simulink model "ROSCO"  (R2023a)
settings: Solver=ode4  StartTime=0.0  StopTime=TMax  FixedStep=simu.dt  RelTol=1e-3  EnableMultiTasking=on
undefined symbols (not defined in the file): A_total, Azimuth_list, B_total, Bd_total, C_total, D_total, Dd_total, DiscIntNeverNeededParam, F, n_FixFrameInputs, n_FixFrameOutputs, n_FixFrameStates2, n_RotTripletInputs, n_RotTripletOutputs, n_RotTripletStates2, new_seq_inp, new_seq_out, new_seq_states, OutList, Parameter, R, rpm2radps, simu, strmatch, uop_total, windspeed_list, wop_total, xop_total, yop_List_total
libraries: simulink x10
(part 2 of 5)

== system ROSCO/LinearModel_Simulink/Transverseu ==
  Azimuth : Inport
  delta_u : Inport  Port=2
  new_seq_inp : Inport  Port=3
  Constant7 : Constant  Value=n_FixFrameInputs
  Constant8 : Constant  Value=n_RotTripletInputs
  MATLAB Function : MATLAB Function  TreatAsAtomicUnit=on
  delta_u_dq : Outport
  wires:
  Constant8/1 -> MATLAB Function/3(n_RotTripletInputs)
  Azimuth/1 -> MATLAB Function/1(Azimuth)
  Constant7/1 -> MATLAB Function/2(n_FixFrameInputs)
  delta_u/1 -> MATLAB Function/4(delta_u)
  new_seq_inp/1 -> MATLAB Function/5(new_seq_inp)
  MATLAB Function/1(delat_u_dq) -> delta_u_dq/1

== system ROSCO/LinearModel_Simulink/uop2uop_dq ==
  Azimuth : Inport
  uop : Inport  Port=2
  Constant1 : Constant  Value=new_seq_inp
  Constant7 : Constant  Value=n_FixFrameInputs
  Constant8 : Constant  Value=n_RotTripletInputs
  MATLAB Function1 : MATLAB Function  TreatAsAtomicUnit=on
  uop_dq : Outport
  wires:
  Constant7/1 -> MATLAB Function1/2(n_FixFrameInputs)
  uop/1 -> MATLAB Function1/4(u)
  MATLAB Function1/1(u_dq) -> uop_dq/1
  Azimuth/1 -> MATLAB Function1/1(Azimuth)
  Constant1/1 -> MATLAB Function1/5(new_seq_inp)
  Constant8/1 -> MATLAB Function1/3(n_RotTripletInputs)

== system ROSCO/LinearModel_Simulink/y_NonLinear ==
  OutData : Inport
  Extract GenSpeed : Fcn  Expr=u(strmatch('GenSpeed',OutList))
  Extract RootMyc1 : Fcn  Expr=u(strmatch('RootMyc1',OutList))
  Extract RootMyc2 : Fcn  Expr=u(strmatch('RootMyc2',OutList))
  Extract RootMyc3 : Fcn  Expr=u(strmatch('RootMyc3',OutList))
  Extract RotSpeed : Fcn  Expr=u(strmatch('RotSpeed',OutList))
  Mux : Mux  Inputs=5
  y_NR : Outport
  wires:
  OutData/1 -> Extract GenSpeed/1, Extract RotSpeed/1, Extract RootMyc2/1, Extract RootMyc3/1, Extract RootMyc1/1
  Extract RootMyc1/1 -> Mux/3
  Mux/1 -> y_NR/1
  Extract RootMyc2/1 -> Mux/4
  Extract RootMyc3/1 -> Mux/5
  Extract GenSpeed/1 -> Mux/1
  Extract RotSpeed/1 -> Mux/2

== system ROSCO/MPC/Extract Azimuth [deg] ==
  OutData : Inport
  Azimut : Scope  NumInputPorts=2
  Extract Azimuth : Fcn  Expr=u(strmatch('Azimuth',OutList))
  Extract RotSpeed : Fcn  Expr=u(strmatch('RotSpeed',OutList))
  Integrator : Integrator
  mod2pi : Fcn  Expr=rem(u, 2*pi)
  rad2deg : Gain  Gain=1/pi*180
  rpm2rad/s : Gain  Gain=pi/30
  Azimuth : Outport
  wires:
  OutData/1 -> Extract RotSpeed/1, Extract Azimuth/1
  rpm2rad/s/1 -> Integrator/1
  mod2pi/1 -> rad2deg/1
  Integrator/1 -> mod2pi/1
  rad2deg/1 -> Azimut/2, Azimuth/1
  Extract RotSpeed/1 -> rpm2rad/s/1
  Extract Azimuth/1 -> Azimut/1

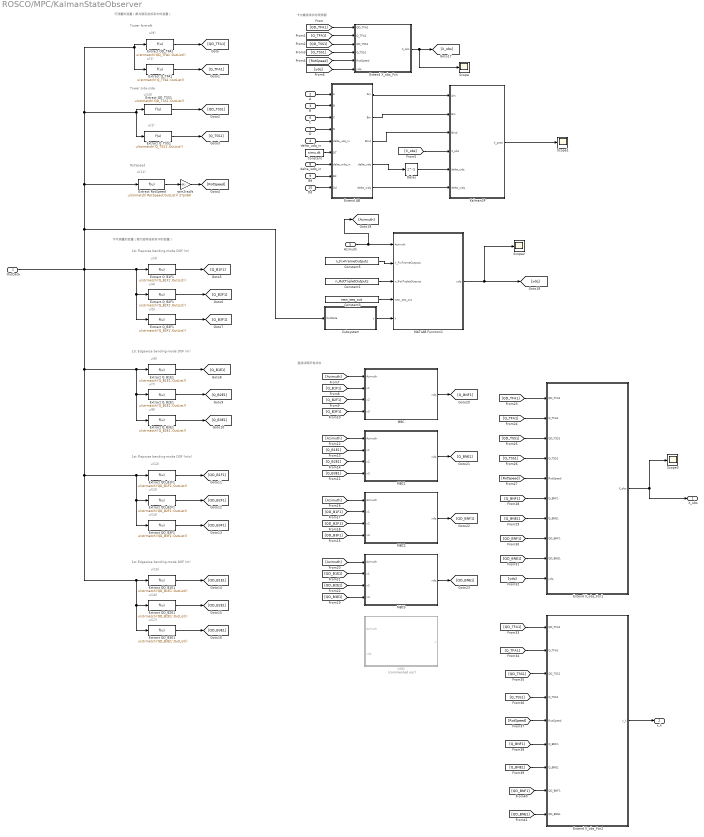
== system ROSCO/MPC/KalmanStateObserver ==
  note: 直接读取所有状态
  note: u(11)
  note: u(2)
  note: u(10)
  note: u(1)
  note: u(9)
  note: 可测量的变量（都为固定坐标系中的变量）
  note: RotSpeed
  note: Tower fore-aft
  note: Tower side-side
  note: 卡尔曼滤波状态观测器
  note: 不可测量的变量（都为旋转坐标系中的变量）
  note: u(3)
  note: u(4)
  note: 1st Flapwise bending-mode DOF (m)
  note: u(5)
  note: u(6)
  note: u(7)
  note: 1st Edgewise bending-mode DOF (m)
  note: u(8)
  note: u(14)
  note: u(12)
  note: u(13)
  note: 1st Flapwise bending-mode DOF (m/s)
  note: 1st Edgewise bending-mode DOF (m)
  note: u(15)
  note: u(17)
  note: u(16)
  OutData : Inport
  A : Inport  Port=2
  B : Inport  Port=3
  delta_udq_in : Inport  Port=4
  Azimuth : Inport  Port=5
  C : Inport  Port=6
  D : Inport  Port=7
  delta_wdq_in : Inport  Port=8
  Bd : Inport  Port=9
  Dd : Inport  Port=10
  Constant : Constant  Value=simu.dt
  Constant1 : Constant  Value=n_RotTripletOutputs
  Constant3 : Constant  Value=new_seq_out
  Constant5 : Constant  Value=n_FixFrameOutputs
  Delay : Delay  DelayLength=1  InitialCondition=0
  Extend AB : MATLAB Function  TreatAsAtomicUnit=on
  Extend X_obs_Fcn : MATLAB Function  TreatAsAtomicUnit=on
  Extend X_obs_Fcn1 : MATLAB Function  TreatAsAtomicUnit=on
  Extend X_obs_Fcn2 : MATLAB Function  TreatAsAtomicUnit=on
  Extract QD_B1E1 : Fcn  Expr=u(strmatch('QD_B1E1',OutList))
  Extract QD_B1F1 : Fcn  Expr=u(strmatch('QD_B1F1',OutList))
  Extract QD_B2E1 : Fcn  Expr=u(strmatch('QD_B2E1',OutList))
  Extract QD_B2F1 : Fcn  Expr=u(strmatch('QD_B2F1',OutList))
  Extract QD_B3E1 : Fcn  Expr=u(strmatch('QD_B3E1',OutList))
  Extract QD_B3F1 : Fcn  Expr=u(strmatch('QD_B3F1',OutList))
  Extract QD_TFA1 : Fcn  Expr=u(strmatch('QD_TFA1',OutList))
  Extract QD_TSS1 : Fcn  Expr=u(strmatch('QD_TSS1',OutList))
  Extract Q_B1E1 : Fcn  Expr=u(strmatch('Q_B1E1',OutList))
  Extract Q_B1F1 : Fcn  Expr=u(strmatch('Q_B1F1',OutList))
  Extract Q_B2E1 : Fcn  Expr=u(strmatch('Q_B2E1',OutList))
  Extract Q_B2F1 : Fcn  Expr=u(strmatch('Q_B2F1',OutList))
  Extract Q_B3E1 : Fcn  Expr=u(strmatch('Q_B3E1',OutList))
  Extract Q_B3F1 : Fcn  Expr=u(strmatch('Q_B3F1',OutList))
  Extract Q_TFA1 : Fcn  Expr=u(strmatch('Q_TFA1',OutList))
  Extract Q_TSS1 : Fcn  Expr=u(strmatch('Q_TSS1',OutList))
  Extract RotSpeed : Fcn  Expr=u(strmatch('RotSpeed',OutList))
  KalmanSP : MATLAB Function  TreatAsAtomicUnit=on
  MATLAB Function1 : MATLAB Function  TreatAsAtomicUnit=on
  MBC : MATLAB Function  TreatAsAtomicUnit=on
  MBC1 : MATLAB Function  TreatAsAtomicUnit=on
  MBC2 : MATLAB Function  TreatAsAtomicUnit=on
  MBC3 : MATLAB Function  TreatAsAtomicUnit=on
  Scope{,1..3} (4 alike) : Scope
  Subsystem : Subsystem
  iMBC : MATLAB Function  Commented=on  TreatAsAtomicUnit=on
  rpm2rad/s : Gain  Gain=2*pi/60
  X_obs : Outport
  x_k : Outport  Port=2
  wires:
  Extract Q_TFA1/1 -> [Q_TFA1]
  Extract QD_TFA1/1 -> [QD_TFA1]
  Extract RotSpeed/1 -> rpm2rad/s/1
  rpm2rad/s/1 -> [RotSpeed]
  Extract QD_TSS1/1 -> [QD_TSS1]
  Extract Q_TSS1/1 -> [Q_TSS1]
  Extract Q_B1F1/1 -> [Q_B1F1]
  Extract Q_B2F1/1 -> [Q_B2F1]
  Extract Q_B3F1/1 -> [Q_B3F1]
  Extract Q_B3E1/1 -> [Q_B3E1]
  Extract Q_B2E1/1 -> [Q_B2E1]
  Extract Q_B1E1/1 -> [Q_B1E1]
  Extract QD_B3F1/1 -> [QD_B3F1]
  Extract QD_B1F1/1 -> [QD_B1F1]
  Extract QD_B2F1/1 -> [QD_B2F1]
  OutData/1 -> Extract QD_TFA1/1, Extract Q_TFA1/1, Extract QD_TSS1/1, Extract Q_TSS1/1, Extract RotSpeed/1, Subsystem/1(OutData), Extract QD_B1E1/1, Extract QD_B2E1/1, Extract QD_B3E1/1, Extract QD_B3F1/1, Extract QD_B2F1/1, Extract QD_B1F1/1, Extract Q_B1E1/1, Extract Q_B2E1/1, Extract Q_B3E1/1, Extract Q_B3F1/1, Extract Q_B2F1/1, Extract Q_B1F1/1
  Extract QD_B3E1/1 -> [QD_B3E1]
  Extract QD_B1E1/1 -> [QD_B1E1]
  Extract QD_B2E1/1 -> [QD_B2E1]
  [QD_TFA1] -> Extend X_obs_Fcn/1(QD_TFA1)
  [Q_TFA1] -> Extend X_obs_Fcn/2(Q_TFA1)
  [QD_TSS1] -> Extend X_obs_Fcn/3(QD_TSS1)
  [Q_TSS1] -> Extend X_obs_Fcn/4(Q_TSS1)
  [RotSpeed] -> Extend X_obs_Fcn/5(RotSpeed)
  Extend X_obs_Fcn/1(X_obs) -> Scope/1, [X_obs]
  [X_obs] -> KalmanSP/4(X_obs)
  Delay/1 -> KalmanSP/5(delta_udq)
  A/1 -> Extend AB/1(A)
  B/1 -> Extend AB/2(B)
  delta_udq_in/1 -> Extend AB/5(delta_udq_in)
  Extend AB/4(delta_udq) -> Delay/1
  Extend AB/2(Bm) -> KalmanSP/2(Bm)
  Extend AB/1(Am) -> KalmanSP/1(Am)
  C/1 -> Extend AB/3(C)
  D/1 -> Extend AB/4(D)
  KalmanSP/1(X_pred) -> Scope1/1
  Subsystem/1(y) -> MATLAB Function1/5(y)
  Constant5/1 -> MATLAB Function1/2(n_FixFrameOutputs)
  Constant1/1 -> MATLAB Function1/3(n_RotTripletOutputs)
  Constant3/1 -> MATLAB Function1/4(new_seq_out)
  Azimuth/1 -> [Azimuth], MATLAB Function1/1(Azimuth)
  MATLAB Function1/1(ydq) -> Scope2/1, [ydq]
  [ydq] -> Extend X_obs_Fcn/6(ydq)
  [Azimuth] -> MBC/1(Azimuth)
  [Q_B1F1] -> MBC/2(x1)
  [Q_B2F1] -> MBC/3(x2)
  [Q_B3F1] -> MBC/4(x3)
  [Q_B3E1] -> MBC1/4(x3)
  [Q_B2E1] -> MBC1/3(x2)
  [Q_B1E1] -> MBC1/2(x1)
  [Azimuth] -> MBC1/1(Azimuth)
  [Azimuth] -> MBC2/1(Azimuth)
  [QD_B1F1] -> MBC2/2(x1)
  [QD_B2F1] -> MBC2/3(x2)
  [QD_B3F1] -> MBC2/4(x3)
  [QD_B3E1] -> MBC3/4(x3)
  [QD_B2E1] -> MBC3/3(x2)
  [QD_B1E1] -> MBC3/2(x1)
  [Azimuth] -> MBC3/1(Azimuth)
  MBC/1(xdq) -> [Q_BNF1]
  MBC1/1(xdq) -> [Q_BNE1]
  MBC2/1(xdq) -> [QD_BNF1]
  MBC3/1(xdq) -> [QD_BNE1]
  [Q_TFA1] -> Extend X_obs_Fcn1/2(Q_TFA1)
  [QD_TSS1] -> Extend X_obs_Fcn1/3(QD_TSS1)
  [RotSpeed] -> Extend X_obs_Fcn1/5(RotSpeed)
  [QD_TFA1] -> Extend X_obs_Fcn1/1(QD_TFA1)
  [Q_TSS1] -> Extend X_obs_Fcn1/4(Q_TSS1)
  [Q_BNF1] -> Extend X_obs_Fcn1/6(Q_BNF1)
  [Q_BNE1] -> Extend X_obs_Fcn1/7(Q_BNE1)
  [QD_BNF1] -> Extend X_obs_Fcn1/8(QD_BNF1)
  [QD_BNE1] -> Extend X_obs_Fcn1/9(QD_BNE1)
  [ydq] -> Extend X_obs_Fcn1/10(ydq)
  Extend X_obs_Fcn1/1(X_obs) -> Scope3/1, X_obs/1
  [QD_TSS1] -> Extend X_obs_Fcn2/3(QD_TSS1)
  [QD_TFA1] -> Extend X_obs_Fcn2/1(QD_TFA1)
  [Q_TSS1] -> Extend X_obs_Fcn2/4(Q_TSS1)
  [QD_BNE1] -> Extend X_obs_Fcn2/9(QD_BNE1)
  [Q_TFA1] -> Extend X_obs_Fcn2/2(Q_TFA1)
  [RotSpeed] -> Extend X_obs_Fcn2/5(RotSpeed)
  [Q_BNF1] -> Extend X_obs_Fcn2/6(Q_BNF1)
  [QD_BNF1] -> Extend X_obs_Fcn2/8(QD_BNF1)
  [Q_BNE1] -> Extend X_obs_Fcn2/7(Q_BNE1)
  Extend X_obs_Fcn2/1(x_k) -> x_k/1
  Constant/1 -> Extend AB/6(DT)
  delta_wdq_in/1 -> Extend AB/7(delta_wdq_in)
  Bd/1 -> Extend AB/8(Bd)
  Dd/1 -> Extend AB/9(Dd)
  Extend AB/3(Bmd) -> KalmanSP/3(Bmd)
  Extend AB/5(delta_wdq) -> KalmanSP/6(delta_wdq)

== system ROSCO/MPC/SwitchOP ==
  WindSpeed : Inport
  MATLAB Function : MATLAB Function  TreatAsAtomicUnit=on
  A : Outport
  B : Outport  Port=2
  C : Outport  Port=3
  D : Outport  Port=4
  yop_list : Outport  Port=5
  xop : Outport  Port=6
  uop : Outport  Port=7
  Bd : Outport  Port=8
  Dd : Outport  Port=9
  wop : Outport  Port=10
  wires:
  WindSpeed/1 -> MATLAB Function/1(windspeed)
  MATLAB Function/1(A) -> A/1
  MATLAB Function/2(B) -> B/1
  MATLAB Function/3(C) -> C/1
  MATLAB Function/4(D) -> D/1
  MATLAB Function/7(yop_list) -> yop_list/1
  MATLAB Function/8(xop) -> xop/1
  MATLAB Function/9(uop) -> uop/1
  MATLAB Function/5(Bd) -> Bd/1
  MATLAB Function/6(Dd) -> Dd/1
  MATLAB Function/10(wop) -> wop/1

== system ROSCO/MPC/Transverseu ==
  Azimuth : Inport
  delta_u : Inport  Port=2
  new_seq_inp : Inport  Port=3
  Constant7 : Constant  Value=n_FixFrameInputs
  Constant8 : Constant  Value=n_RotTripletInputs
  MATLAB Function : MATLAB Function  TreatAsAtomicUnit=on
  delta_u_dq : Outport
  wires:
  Constant8/1 -> MATLAB Function/3(n_RotTripletInputs)
  Azimuth/1 -> MATLAB Function/1(Azimuth)
  Constant7/1 -> MATLAB Function/2(n_FixFrameInputs)
  delta_u/1 -> MATLAB Function/4(delta_u)
  new_seq_inp/1 -> MATLAB Function/5(new_seq_inp)
  MATLAB Function/1(delat_u_dq) -> delta_u_dq/1

== system ROSCO/MPC/y_NonLinear ==
  OutData : Inport
  Extract GenSpeed : Fcn  Expr=u(strmatch('GenSpeed',OutList))
  Extract RootMyc1 : Fcn  Expr=u(strmatch('RootMyc1',OutList))
  Extract RootMyc2 : Fcn  Expr=u(strmatch('RootMyc2',OutList))
  Extract RootMyc3 : Fcn  Expr=u(strmatch('RootMyc3',OutList))
  Extract RotSpeed : Fcn  Expr=u(strmatch('RotSpeed',OutList))
  Mux : Mux  Inputs=5
  y_NR : Outport
  wires:
  OutData/1 -> Extract GenSpeed/1, Extract RotSpeed/1, Extract RootMyc2/1, Extract RootMyc3/1, Extract RootMyc1/1
  Extract RootMyc1/1 -> Mux/3
  Mux/1 -> y_NR/1
  Extract RootMyc2/1 -> Mux/4
  Extract RootMyc3/1 -> Mux/5
  Extract GenSpeed/1 -> Mux/1
  Extract RotSpeed/1 -> Mux/2

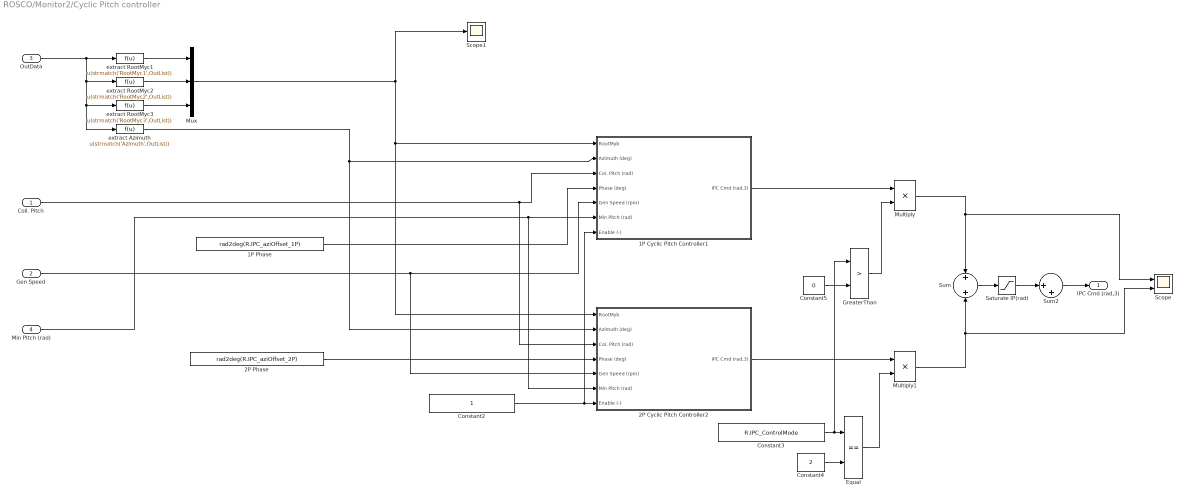
== system ROSCO/Monitor2/Cyclic Pitch controller ==
  Coll. Pitch : Inport
  Gen Speed : Inport  Port=2
  OutData : Inport  Port=3
  Min PItch (rad) : Inport  Port=4
  1P Cyclic Pitch Controller1 : Subsystem
  1P Phase : Constant  Value=rad2deg(R.IPC_aziOffset_1P)
  2P Cyclic Pitch Controller2 : Subsystem
  2P Phase : Constant  Value=rad2deg(R.IPC_aziOffset_2P)
  Constant2 : Constant
  Constant3 : Constant  Value=R.IPC_ControlMode
  Constant4 : Constant  Value=2
  Constant5 : Constant  Value=0
  Equal : RelationalOperator  Operator===  OutDataTypeStr=boolean  RndMeth=Simplest  InputSameDT=off
  GreaterThan : RelationalOperator  Operator=>  OutDataTypeStr=boolean  RndMeth=Simplest  InputSameDT=off
  Multiply : Product
  Multiply1 : Product
  Mux : Mux  Inputs=3
  Saturate IP(rad) : Saturate  UpperLimit=0.052  LowerLimit=-0.052
  Scope : Scope  NumInputPorts=2
  Scope1 : Scope
  Sum : Sum  Inputs=+|+
  Sum2 : Sum  Inputs=|++
  extract Azimuth : Fcn  Expr=u(strmatch('Azimuth',OutList))
  extract RootMyc1 : Fcn  Expr=u(strmatch('RootMyc1',OutList))
  extract RootMyc2 : Fcn  Expr=u(strmatch('RootMyc2',OutList))
  extract RootMyc3 : Fcn  Expr=u(strmatch('RootMyc3',OutList))
  IPC Cmd (rad,3) : Outport  VectorParamsAs1DForOutWhenUnconnected=off
  wires:
  1P Phase/1 -> 1P Cyclic Pitch Controller1/4(Phase (deg))
  Coll. Pitch/1 -> 2P Cyclic Pitch Controller2/3(Col. Pitch (rad)), 1P Cyclic Pitch Controller1/3(Col. Pitch (rad))
  Gen Speed/1 -> 2P Cyclic Pitch Controller2/5(Gen Speed (rpm)), 1P Cyclic Pitch Controller1/5(Gen Speed (rpm))
  1P Cyclic Pitch Controller1/1(IPC Cmd (rad,3)) -> Multiply/1
  Mux/1 -> Scope1/1, 1P Cyclic Pitch Controller1/1(RootMyb), 2P Cyclic Pitch Controller2/1(RootMyb)
  extract Azimuth/1 -> 2P Cyclic Pitch Controller2/2(Azimuth (deg)), 1P Cyclic Pitch Controller1/2(Azimuth (deg))
  Min PItch (rad)/1 -> 2P Cyclic Pitch Controller2/6(Min Pitch (rad)), 1P Cyclic Pitch Controller1/6(Min Pitch (rad))
  2P Phase/1 -> 2P Cyclic Pitch Controller2/4(Phase (deg))
  2P Cyclic Pitch Controller2/1(IPC Cmd (rad,3)) -> Multiply1/1
  Multiply1/1 -> Scope/2, Sum/2
  Multiply/1 -> Sum/1, Scope/1
  Sum/1 -> Saturate IP(rad)/1
  Sum2/1 -> IPC Cmd (rad,3)/1
  Constant2/1 -> 1P Cyclic Pitch Controller1/7(Enable (-)), 2P Cyclic Pitch Controller2/7(Enable (-))
  Constant4/1 -> Equal/2
  Equal/1 -> Multiply1/2
  Constant3/1 -> GreaterThan/1, Equal/1
  Constant5/1 -> GreaterThan/2
  GreaterThan/1 -> Multiply/2
  extract RootMyc2/1 -> Mux/2
  extract RootMyc3/1 -> Mux/3
  OutData/1 -> extract RootMyc1/1, extract RootMyc2/1, extract Azimuth/1, extract RootMyc3/1
  extract RootMyc1/1 -> Mux/1
  Saturate IP(rad)/1 -> Sum2/1

== system ROSCO/PitchSaturation/Integral ==
  x : Inport
  Gain : Inport  Port=2
  Gain1 : Gain  Gain=simu.dt
  Maximum Pitch : Constant  Value=100
  Minimum Pitch : Constant  Value=-100
  Multiply : Product
  Saturate Integral Term : simulink/Discontinuities/Saturation Dynamic  OutMin=[]  OutMax=[]  OutDataTypeStr=Inherit: Same as second input  OutDataType=fixdt(1, 16)  OutScaling=2^-10  RndMeth=Nearest  DoSatur=off
  Scope : Scope  NumInputPorts=2
  Sum : Sum  Inputs=|++
  Unit Delay : UnitDelay  SampleTime=-1  HasFrameUpgradeWarning=on
  Int x : Outport  VectorParamsAs1DForOutWhenUnconnected=off
  wires:
  Maximum Pitch/1 -> Saturate Integral Term/1
  Unit Delay/1 -> Sum/2
  Minimum Pitch/1 -> Saturate Integral Term/3
  Sum/1 -> Saturate Integral Term/2
  x/1 -> Scope/1, Gain1/1
  Gain/1 -> Multiply/2
  Saturate Integral Term/1 -> Scope/2, Int x/1, Unit Delay/1
  Gain1/1 -> Multiply/1
  Multiply/1 -> Sum/1

== system ROSCO/SetpointSmoother/Filter Delta_GenRef ==
  GainBias : Inport
  Discrete Filter : DiscreteFilter  Numerator=F.F_SS.b  Denominator=F.F_SS.a
  GainBiasF : Outport  VectorParamsAs1DForOutWhenUnconnected=off
  wires:
  Discrete Filter/1 -> GainBiasF/1
  GainBias/1 -> Discrete Filter/1

== system ROSCO/Torque Controller/Integral ==
  SpeedErr : Inport
  Gain : Inport  Port=2
  Gain1 : Gain  Gain=simu.dt
  Maximum Torque : Constant  Value=R.VS_RtTq
  Minimum Torque : Constant  Value=0
  Multiply : Product
  Saturate Integral Term : simulink/Discontinuities/Saturation Dynamic  OutMin=[]  OutMax=[]  OutDataTypeStr=Inherit: Same as second input  OutDataType=fixdt(1, 16)  OutScaling=2^-10  RndMeth=Nearest  DoSatur=off
  Sum : Sum  Inputs=|++
  Unit Delay : UnitDelay  InitialCondition=R.VS_RtTq  SampleTime=-1  HasFrameUpgradeWarning=on
  IntSpdErr : Outport  VectorParamsAs1DForOutWhenUnconnected=off
  wires:
  Maximum Torque/1 -> Saturate Integral Term/1
  Unit Delay/1 -> Sum/2
  Minimum Torque/1 -> Saturate Integral Term/3
  Sum/1 -> Saturate Integral Term/2
  SpeedErr/1 -> Gain1/1
  Gain/1 -> Multiply/2
  Saturate Integral Term/1 -> IntSpdErr/1, Unit Delay/1
  Gain1/1 -> Multiply/1
  Multiply/1 -> Sum/1

== system ROSCO/Torque Controller/VS_OmegaRef ==
  WindSpeedEst : Inport
  Omega_opt : Subsystem
  Reference TSR : Constant  Value=R.VS_TSRopt
  Saturation : Saturate  UpperLimit=R.PC_RefSpd  LowerLimit=R.VS_MinOMSpd
  To Workspace1 : ToWorkspace  VariableName=Om_opt  SaveFormat=Timeseries  SampleTime=-1
  VS_OmegaOpt : Outport  VectorParamsAs1DForOutWhenUnconnected=off
  wires:
  WindSpeedEst/1 -> Omega_opt/2(Wind Speed)
  Omega_opt/1(Omega_opt) -> Saturation/1
  Reference TSR/1 -> Omega_opt/1(TSR_opt)
  Saturation/1 -> VS_OmegaOpt/1, To Workspace1/1

== system ROSCO/Wind Speed Estimator/WE_Params ==
  Constant1 : Constant  Value=R.WE_Jtot
  Constant2 : Constant  Value=R.WE_RhoAir
  Constant3 : Constant  Value=R.WE_BladeRadius
  Constant4 : Constant  Value=R.WE_GearboxRatio
  Mux : Mux
  WE_Params : Outport
  wires:
  Constant2/1 -> Mux/2
  Mux/1 -> WE_Params/1
  Constant4/1 -> Mux/4
  Constant1/1 -> Mux/1
  Constant3/1 -> Mux/3

== system ROSCO/LinearModel_Simulink/KalmanStateObserver/Subsystem ==
  OutData : Inport
  Extract GenSpeed : Fcn  Expr=u(strmatch('GenSpeed',OutList))
  Extract RootMyc1 : Fcn  Expr=u(strmatch('RootMyc1',OutList))
  Extract RootMyc2 : Fcn  Expr=u(strmatch('RootMyc2',OutList))
  Extract RootMyc3 : Fcn  Expr=u(strmatch('RootMyc3',OutList))
  Extract RotSpeed : Fcn  Expr=u(strmatch('RotSpeed',OutList))
  Mux : Mux  Inputs=5
  y : Outport
  wires:
  Extract GenSpeed/1 -> Mux/1
  OutData/1 -> Extract GenSpeed/1, Extract RotSpeed/1, Extract RootMyc2/1, Extract RootMyc3/1, Extract RootMyc1/1
  Mux/1 -> y/1
  Extract RotSpeed/1 -> Mux/2
  Extract RootMyc1/1 -> Mux/3
  Extract RootMyc2/1 -> Mux/4
  Extract RootMyc3/1 -> Mux/5

== system ROSCO/MPC/KalmanStateObserver/Subsystem ==
  OutData : Inport
  Extract GenSpeed : Fcn  Expr=u(strmatch('GenSpeed',OutList))
  Extract RootMyc1 : Fcn  Expr=u(strmatch('RootMyc1',OutList))
  Extract RootMyc2 : Fcn  Expr=u(strmatch('RootMyc2',OutList))
  Extract RootMyc3 : Fcn  Expr=u(strmatch('RootMyc3',OutList))
  Extract RotSpeed : Fcn  Expr=u(strmatch('RotSpeed',OutList))
  Mux : Mux  Inputs=5
  y : Outport
  wires:
  Extract GenSpeed/1 -> Mux/1
  OutData/1 -> Extract GenSpeed/1, Extract RotSpeed/1, Extract RootMyc2/1, Extract RootMyc3/1, Extract RootMyc1/1
  Mux/1 -> y/1
  Extract RotSpeed/1 -> Mux/2
  Extract RootMyc1/1 -> Mux/3
  Extract RootMyc2/1 -> Mux/4
  Extract RootMyc3/1 -> Mux/5

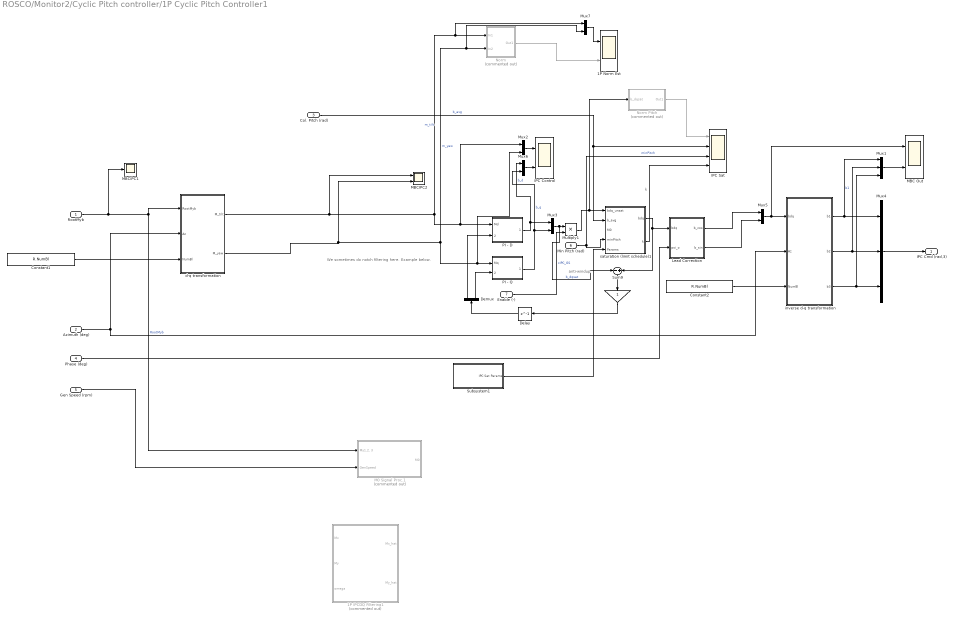
== system ROSCO/Monitor2/Cyclic Pitch controller/1P Cyclic Pitch Controller1 ==
  note: We sometimes do notch filtering here. Example below.
  note: k
  note: anti-windup
  RootMyb : Inport
  Azimuth (deg) : Inport  Port=2
  Col. Pitch (rad) : Inport  Port=3
  Phase (deg) : Inport  Port=4
  Gen Speed (rpm) : Inport  Port=5
  Min Pitch (rad) : Inport  Port=6
  Enable (-) : Inport  Port=7
  " " : Gain
  1P IPCDQ Filtering1 : Subsystem  Commented=on
  1P Norm Est : Scope  NumInputPorts=2
  Constant1 : Constant  Value=R.NumBl
  Constant2 : Constant  Value=R.NumBl
  Delay : Delay  DelayLength=1
  Demux : Demux  Outputs=2
  IPC Control : Scope  NumInputPorts=2
  IPC Sat : Scope  NumInputPorts=4
  Lead Correction : MATLAB Function  TreatAsAtomicUnit=on
  M0 Signal Proc.1 : Subsystem  Commented=on
  MBC Out : Scope  NumInputPorts=2
  MBCIPC1 : Scope
  MBCIPC2 : Scope  NumInputPorts=2
  Multiply1 : Product
  Mux1 : Mux  Inputs=3
  Mux{2..3,5..7} (5 alike) : Mux  Inputs=2
  Mux4 : Mux  Inputs=3
  Norm : Subsystem  Commented=on
  Norm Pitch : Subsystem  Commented=on
  PI - D : Subsystem  TreatAsAtomicUnit=on  SystemSampleTime=simu.dt
      settings: MinAlgLoopOccurrences=on
  PI - Q : Subsystem  TreatAsAtomicUnit=on  SystemSampleTime=simu.dt
      settings: MinAlgLoopOccurrences=on
  Subsystem1 : Subsystem
  Sum9 : Sum  Inputs=-|+
  d-q transformation : MATLAB Function  TreatAsAtomicUnit=on
  inverse d-q transformation : MATLAB Function  TreatAsAtomicUnit=on
  saturation (limit schedule)1 : MATLAB Function  TreatAsAtomicUnit=on
  IPC Cmd (rad,3) : Outport  VectorParamsAs1DForOutWhenUnconnected=off
  wires:
  Col. Pitch (rad)/1 -> saturation (limit schedule)1/2(b_avg), IPC Sat/2  "b_avg"
  saturation (limit schedule)1/1(bdq) -> Sum9/2, Lead Correction/1(bdq)
  Gen Speed (rpm)/1 -> M0 Signal Proc.1/2(GenSpeed)
  d-q transformation/1(M_tilt) -> Mux2/1, PI - D/1(Md), Mux7/1, Norm/1(In1), MBCIPC2/1  "m_tilt"
  Mux5/1 -> MBC Out/1, inverse d-q transformation/1(bdq)
  inverse d-q transformation/3(b3) -> Mux1/3, Mux4/3
  Phase (deg)/1 -> Lead Correction/2(psi_o)
  PI - Q/1(Theta_yaw) -> Mux6/2, Mux3/2  "b_q"
  PI - D/1(Theta_tilt) -> Mux3/1, Mux6/1  "b_d"
  Demux/1 -> PI - D/2(Anti-windup)
  inverse d-q transformation/1(b1) -> Mux1/1, Mux4/1  "b1"
  Demux/2 -> PI - Q/2(Anti-windup)
  inverse d-q transformation/2(b2) -> Mux1/2, Mux4/2
  Mux4/1 -> IPC Cmd (rad,3)/1
  Delay/1 -> Demux/1
  " "/1 -> Delay/1
  RootMyb/1 -> M0 Signal Proc.1/1("My1,2, 3"), d-q transformation/1(RootMyb), MBCIPC1/1  "RootMyb"
  Sum9/1 -> " "/1
  Azimuth (deg)/1 -> d-q transformation/2(Az), inverse d-q transformation/2(Az)
  Lead Correction/1(b_cos) -> Mux5/1
  Lead Correction/2(b_sin) -> Mux5/2
  saturation (limit schedule)1/2(k) -> IPC Sat/4
  Constant1/1 -> d-q transformation/3(NumBl)
  Constant2/1 -> inverse d-q transformation/3(NumBl)
  d-q transformation/2(M_yaw) -> Mux2/2, PI - Q/1(Mq), Mux7/2, Norm/2(In2), MBCIPC2/2  "m_yaw"
  Mux1/1 -> MBC Out/2
  Mux6/1 -> IPC Control/2
  Mux2/1 -> IPC Control/1
  Mux7/1 -> 1P Norm Est/1
  Norm/1(Out1) -> 1P Norm Est/2
  Min Pitch (rad)/1 -> IPC Sat/3, saturation (limit schedule)1/4(minPitch)  "minPitch"
  Norm Pitch/1(Out1) -> IPC Sat/1
  Enable (-)/1 -> Multiply1/2  "cIPC_GS"
  Subsystem1/1(IPC Sat Params) -> saturation (limit schedule)1/5(Params)
  Mux3/1 -> Sum9/1, Multiply1/1  "b_dqsat"
  Multiply1/1 -> Norm Pitch/1(b_dqsat), saturation (limit schedule)1/1(bdq_unsat)
  ? -> 1P IPCDQ Filtering1/2(My)  "m_yaw"

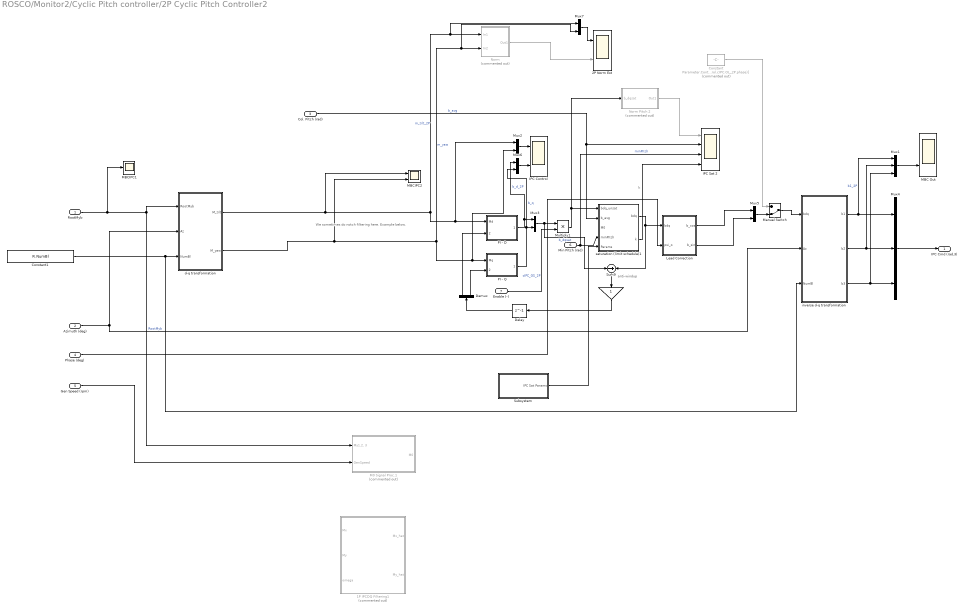
== system ROSCO/Monitor2/Cyclic Pitch controller/2P Cyclic Pitch Controller2 ==
  note: We sometimes do notch filtering here. Example below.
  note: anti-windup
  note: k
  RootMyb : Inport
  Azimuth (deg) : Inport  Port=2
  Col. Pitch (rad) : Inport  Port=3
  Phase (deg) : Inport  Port=4
  Gen Speed (rpm) : Inport  Port=5
  Min Pitch (rad) : Inport  Port=6
  Enable (-) : Inport  Port=7
  " " : Gain
  1P IPCDQ Filtering1 : Subsystem  Commented=on
  2P Norm Est : Scope  NumInputPorts=2
  Constant : Constant  Commented=on  Value=Parameter.Control.cIPC.OL_2P.amp * [cosd(Parameter.Control.cIPC.OL_2P.phase), sind(Parameter.Control.cIPC.OL_2P.phase)]
  Constant1 : Constant  Value=R.NumBl
  Delay : Delay  DelayLength=1
  Demux : Demux  Outputs=2
  IPC Control : Scope  NumInputPorts=2
  IPC Sat 2 : Scope  NumInputPorts=4
  Lead Correction : MATLAB Function  TreatAsAtomicUnit=on
  M0 Signal Proc.1 : Subsystem  Commented=on
  MBC Out : Scope  NumInputPorts=2
  MBCIPC1 : Scope
  MBCIPC2 : Scope  NumInputPorts=2
  Manual Switch : ManualSwitch  CurrentSetting=0
  Multiply1 : Product
  Mux1 : Mux  Inputs=3
  Mux{2..3,5..7} (5 alike) : Mux  Inputs=2
  Mux4 : Mux  Inputs=3
  Norm : Subsystem  Commented=on
  Norm Pitch 2 : Subsystem  Commented=on
  PI - D : Subsystem  TreatAsAtomicUnit=on  SystemSampleTime=simu.dt
      settings: MinAlgLoopOccurrences=on
  PI - Q : Subsystem  TreatAsAtomicUnit=on  SystemSampleTime=simu.dt
      settings: MinAlgLoopOccurrences=on
  Subsystem : Subsystem
  Sum9 : Sum  Inputs=-|+
  d-q transformation : MATLAB Function  TreatAsAtomicUnit=on
  inverse d-q transformation : MATLAB Function  TreatAsAtomicUnit=on
  saturation (limit schedule)1 : MATLAB Function  TreatAsAtomicUnit=on
  IPC Cmd (rad,3) : Outport  VectorParamsAs1DForOutWhenUnconnected=off
  wires:
  Enable (-)/1 -> Multiply1/2  "cIPC_GS_2P"
  Norm Pitch 2/1(Out1) -> IPC Sat 2/1
  Min Pitch (rad)/1 -> saturation (limit schedule)1/4(minPitch), IPC Sat 2/3  "minPitch"
  Norm/1(Out1) -> 2P Norm Est/2
  Mux7/1 -> 2P Norm Est/1
  Mux2/1 -> IPC Control/1
  Mux6/1 -> IPC Control/2
  Mux1/1 -> MBC Out/2
  d-q transformation/2(M_yaw) -> PI - Q/1(Mq), Mux2/2, Norm/2(In2), Mux7/2, MBCIPC2/2  "m_yaw"
  Constant1/1 -> inverse d-q transformation/3(NumBl), d-q transformation/3(NumBl)
  saturation (limit schedule)1/2(k) -> IPC Sat 2/4
  Lead Correction/2(b_sin) -> Mux5/2
  Lead Correction/1(b_cos) -> Mux5/1
  Azimuth (deg)/1 -> inverse d-q transformation/2(Az), d-q transformation/2(Az)
  Sum9/1 -> " "/1
  RootMyb/1 -> MBCIPC1/1, M0 Signal Proc.1/1("My1,2, 3"), d-q transformation/1(RootMyb)  "RootMyb"
  " "/1 -> Delay/1
  Delay/1 -> Demux/1
  Mux4/1 -> IPC Cmd (rad,3)/1
  inverse d-q transformation/2(b2) -> Mux4/2, Mux1/2
  Demux/2 -> PI - Q/2(Anti-windup)
  inverse d-q transformation/1(b1) -> Mux4/1, Mux1/1  "b1_2P"
  Demux/1 -> PI - D/2(Anti-windup)
  PI - D/1(Theta_tilt) -> Mux6/1, Mux3/1  "b_d_2P"
  PI - Q/1(Theta_yaw) -> Mux6/2, Mux3/2  "b_q"
  Phase (deg)/1 -> Lead Correction/2(psi_o)
  inverse d-q transformation/3(b3) -> Mux4/3, Mux1/3
  d-q transformation/1(M_tilt) -> PI - D/1(Md), Mux2/1, Norm/1(In1), Mux7/1, MBCIPC2/1  "m_tilt_2P"
  Gen Speed (rpm)/1 -> M0 Signal Proc.1/2(GenSpeed)
  saturation (limit schedule)1/1(bdq) -> Lead Correction/1(bdq), Sum9/2
  Col. Pitch (rad)/1 -> IPC Sat 2/2, saturation (limit schedule)1/2(b_avg)  "b_avg"
  Subsystem/1(IPC Sat Params) -> saturation (limit schedule)1/5(Params)
  Mux3/1 -> Sum9/1, Multiply1/1  "b_dqsat"
  Multiply1/1 -> Norm Pitch 2/1(b_dqsat), saturation (limit schedule)1/1(bdq_unsat)
  Mux5/1 -> Manual Switch/2
  Manual Switch/1 -> inverse d-q transformation/1(bdq)
  Constant/1 -> Manual Switch/1

== system ROSCO/Torque Controller/VS_OmegaRef/Omega_opt ==
  note: % Assuming known wind speed, initially, and not using GenSpeed
  TSR_opt : Inport
  Wind Speed : Inport  Port=2
  Divide : Product  Inputs=*/
  Multiply : Product
  "Rot -> GenSpeed" : Gain  Gain=R.GBRatio
  Rotor Radius : Constant  Value=R.RotorRad
  Omega_opt : Outport  VectorParamsAs1DForOutWhenUnconnected=off
  wires:
  TSR_opt/1 -> Multiply/1
  Wind Speed/1 -> Multiply/2
  Multiply/1 -> Divide/1
  Rotor Radius/1 -> Divide/2
  Divide/1 -> "Rot -> GenSpeed"/1
  "Rot -> GenSpeed"/1 -> Omega_opt/1

== system ROSCO/Monitor2/Cyclic Pitch controller/1P Cyclic Pitch Controller1/1P IPCDQ Filtering1 ==
  Mx : Inport
  My : Inport  Port=2
  omega : Inport  Port=3
  Discrete Filter2 : DiscreteFilter  Numerator=Parameter.Control.cIPC.IPCDQ_LPF.Numerator{1}  Denominator=Parameter.Control.cIPC.IPCDQ_LPF.Denominator{1}  SampleTime=Parameter.Control.DT
  Discrete Filter3 : DiscreteFilter  Numerator=Parameter.Control.cIPC.IPCDQ_LPF.Numerator{1}  Denominator=Parameter.Control.cIPC.IPCDQ_LPF.Denominator{1}  SampleTime=Parameter.Control.DT
  IPC NFs Man 2 : Scope  NumInputPorts=2
  Moving 3P Notch Man Y : Subsystem
  Moving 3P Notch Man Z : Subsystem
  Moving 6P Notch Man Y : Subsystem
  Moving 6P Notch Man Z : Subsystem
  Mux : Mux  Inputs=2
  Mux1 : Mux  Inputs=2
  Mx_hat : Outport  VectorParamsAs1DForOutWhenUnconnected=off
  My_hat : Outport  Port=2  VectorParamsAs1DForOutWhenUnconnected=off
  wires:
  omega/1 -> Moving 6P Notch Man Y/2(GenSpeedIN), Moving 3P Notch Man Y/2(GenSpeedIN), Moving 6P Notch Man Z/2(GenSpeedIN), Moving 3P Notch Man Z/2(GenSpeedIN)
  Mx/1 -> Mux/1, Moving 3P Notch Man Y/1(Input)
  My/1 -> Mux1/1, Moving 3P Notch Man Z/1(Input)
  Moving 6P Notch Man Z/1(Output) -> Discrete Filter3/1
  Moving 6P Notch Man Y/1(Output) -> Discrete Filter2/1
  Moving 3P Notch Man Y/1(Output) -> Moving 6P Notch Man Y/1(Input)
  Moving 3P Notch Man Z/1(Output) -> Moving 6P Notch Man Z/1(Input)
  Mux1/1 -> IPC NFs Man 2/2
  Mux/1 -> IPC NFs Man 2/1
  Discrete Filter3/1 -> Mux1/2, My_hat/1
  Discrete Filter2/1 -> Mux/2, Mx_hat/1

== system ROSCO/Monitor2/Cyclic Pitch controller/1P Cyclic Pitch Controller1/M0 Signal Proc.1 ==
  "My1,2, 3" : Inport
  GenSpeed : Inport  Port=2
  Add : Sum  Inputs=+++
  Demux1 : Demux  Outputs=3
  Discrete Filter : DiscreteFilter  Numerator=Parameter.Control.cIPC.PSM0_LPF.Numerator{1}  Denominator=Parameter.Control.cIPC.PSM0_LPF.Denominator{1}  a0EqualsOne=on
  Gain : Gain  Gain=1/3
  Moving 1P Notch Man : Subsystem
  Moving 3P Notch Man : Subsystem
  Mux : Mux  Inputs=2
  Scope : Scope  NumInputPorts=2
  M0 : Outport  VectorParamsAs1DForOutWhenUnconnected=off
  wires:
  Demux1/1 -> Add/1
  Demux1/2 -> Add/2
  Add/1 -> Gain/1
  "My1,2, 3"/1 -> Demux1/1
  GenSpeed/1 -> Moving 3P Notch Man/2(GenSpeedIN), Moving 1P Notch Man/2(GenSpeedIN)
  Demux1/3 -> Add/3
  Moving 1P Notch Man/1(Output) -> Moving 3P Notch Man/1(Input)
  Mux/1 -> Scope/2
  Gain/1 -> Scope/1, Moving 1P Notch Man/1(Input)
  Moving 3P Notch Man/1(Output) -> Discrete Filter/1
  Discrete Filter/1 -> Mux/1, M0/1

== system ROSCO/Monitor2/Cyclic Pitch controller/1P Cyclic Pitch Controller1/Norm ==
  In1 : Inport
  In2 : Inport  Port=2
  Add : Sum
  Discrete Filter1 : DiscreteFilter  Numerator=Parameter.Control.cIPC.IPCDQ_LPF.num{1}  Denominator=Parameter.Control.cIPC.IPCDQ_LPF.den{1}  SampleTime=Parameter.Control.DT
  Product : Product
  Product1 : Product
  Sqrt : Sqrt
  Out1 : Outport  VectorParamsAs1DForOutWhenUnconnected=off
  wires:
  Product/1 -> Add/1
  Product1/1 -> Add/2
  Sqrt/1 -> Discrete Filter1/1
  Add/1 -> Sqrt/1
  In2/1 -> Product1/1, Product1/2
  In1/1 -> Product/1, Product/2
  Discrete Filter1/1 -> Out1/1

== system ROSCO/Monitor2/Cyclic Pitch controller/1P Cyclic Pitch Controller1/Norm Pitch ==
  b_dqsat : Inport
  Demux1 : Demux  Outputs=2
  Sqrt : Sqrt
  Square : Math  Operator=square  SignedPower=on
  Square1 : Math  Operator=square  SignedPower=on
  Sum : Sum
  Out1 : Outport  VectorParamsAs1DForOutWhenUnconnected=off
  wires:
  Demux1/1 -> Square/1
  Square1/1 -> Sum/2
  b_dqsat/1 -> Demux1/1
  Sum/1 -> Sqrt/1
  Demux1/2 -> Square1/1
  Square/1 -> Sum/1
  Sqrt/1 -> Out1/1

== system ROSCO/Monitor2/Cyclic Pitch controller/1P Cyclic Pitch Controller1/PI - D ==
  Md : Inport
  Anti-windup : Inport  Port=2
  Discrete Derivative : simulink/Discrete/Discrete Derivative  gainval=1.0  ICPrevScaledInput=0.0  OutMin=[]  OutMax=[]  OutDataType=fixdt(1, 16)  OutScaling=2^-10  DoSatur=off
  Discrete Filter1 : DiscreteFilter  Commented=through  Numerator=Parameter.Control.cIPC.IPCDQ_LPF.num{1}  Denominator=Parameter.Control.cIPC.IPCDQ_LPF.den{1}  SampleTime=Parameter.Control.DT
  Integrator : DiscreteIntegrator  IntegratorMethod=Integration: Backward Euler  gainval=1  SampleTime=simu.dt  UpperSaturationLimit=1.570796/(.008068634/9.5492966)/(1./(1.+pi/2/.109997))  LowerSaturationLimit=0  ICPrevOutput=DiscIntNeverNeededParam  ICPrevScaledInput=DiscIntNeverNeededParam
  Kd : Gain  Gain=0
  Ki : Gain  Gain=R.IPC_KI_2P
  Kp : Gain  Gain=R.IPC_KP_1P
  Scope : Scope  NumInputPorts=2
  Sum3 : Sum  Inputs=+++
  Sum8 : Sum  Inputs=|++
  Theta_tilt : Outport  VectorParamsAs1DForOutWhenUnconnected=off
  wires:
  Ki/1 -> Sum8/1
  Sum3/1 -> Scope/1, Theta_tilt/1
  Md/1 -> Ki/1, Kp/1, Discrete Filter1/1
  Anti-windup/1 -> Scope/2, Sum8/2
  Sum8/1 -> Integrator/1
  Kd/1 -> Discrete Derivative/1
  Kp/1 -> Sum3/2
  Discrete Derivative/1 -> Sum3/1
  Integrator/1 -> Sum3/3
  Discrete Filter1/1 -> Kd/1

== system ROSCO/Monitor2/Cyclic Pitch controller/1P Cyclic Pitch Controller1/PI - Q ==
  Mq : Inport
  Anti-windup : Inport  Port=2
  Discrete Derivative : simulink/Discrete/Discrete Derivative  gainval=1.0  ICPrevScaledInput=0.0  OutMin=[]  OutMax=[]  OutDataType=fixdt(1, 16)  OutScaling=2^-10  DoSatur=off
  Discrete Filter1 : DiscreteFilter  Commented=through  Numerator=Parameter.Control.cIPC.IPCDQ_LPF.num{1}  Denominator=Parameter.Control.cIPC.IPCDQ_LPF.den{1}  SampleTime=Parameter.Control.DT
  Integrator1 : DiscreteIntegrator  IntegratorMethod=Integration: Backward Euler  gainval=1  SampleTime=simu.dt  UpperSaturationLimit=1.570796/(.008068634/9.5492966)/(1./(1.+pi/2/.109997))  LowerSaturationLimit=0  ICPrevOutput=DiscIntNeverNeededParam  ICPrevScaledInput=DiscIntNeverNeededParam
  Kd : Gain  Gain=0
  Ki : Gain  Gain=R.IPC_KI_1P
  Kp : Gain  Gain=R.IPC_KP_1P
  Sum10 : Sum  Inputs=|++
  Sum3 : Sum  Inputs=+++
  Theta_yaw : Outport  VectorParamsAs1DForOutWhenUnconnected=off
  wires:
  Sum3/1 -> Theta_yaw/1
  Sum10/1 -> Integrator1/1
  Anti-windup/1 -> Sum10/2
  Integrator1/1 -> Sum3/3
  Ki/1 -> Sum10/1
  Kp/1 -> Sum3/2
  Mq/1 -> Discrete Filter1/1, Kp/1, Ki/1
  Kd/1 -> Discrete Derivative/1
  Discrete Derivative/1 -> Sum3/1
  Discrete Filter1/1 -> Kd/1

== system ROSCO/Monitor2/Cyclic Pitch controller/1P Cyclic Pitch Controller1/Subsystem1 ==
  Constant3 : Constant
  Constant4 : Constant  Value=0
  Constant5 : Constant  Value=0
  Mux : Mux  Inputs=3
  IPC Sat Params : Outport  VectorParamsAs1DForOutWhenUnconnected=off
  wires:
  Constant3/1 -> Mux/1
  Constant4/1 -> Mux/2
  Constant5/1 -> Mux/3
  Mux/1 -> IPC Sat Params/1

== system ROSCO/Monitor2/Cyclic Pitch controller/2P Cyclic Pitch Controller2/1P IPCDQ Filtering1 ==
  Mx : Inport
  My : Inport  Port=2
  omega : Inport  Port=3
  Discrete Filter2 : DiscreteFilter  Numerator=Parameter.Control.cIPC.IPCDQ_LPF.Numerator{1}  Denominator=Parameter.Control.cIPC.IPCDQ_LPF.Denominator{1}  SampleTime=Parameter.Control.DT
  Discrete Filter3 : DiscreteFilter  Numerator=Parameter.Control.cIPC.IPCDQ_LPF.Numerator{1}  Denominator=Parameter.Control.cIPC.IPCDQ_LPF.Denominator{1}  SampleTime=Parameter.Control.DT
  IPC NFs Man 2 : Scope  NumInputPorts=2
  Moving 3P Notch Man Y : Subsystem
  Moving 3P Notch Man Z : Subsystem
  Moving 6P Notch Man Y : Subsystem
  Moving 6P Notch Man Z : Subsystem
  Mux : Mux  Inputs=2
  Mux1 : Mux  Inputs=2
  Mx_hat : Outport  VectorParamsAs1DForOutWhenUnconnected=off
  My_hat : Outport  Port=2  VectorParamsAs1DForOutWhenUnconnected=off
  wires:
  omega/1 -> Moving 6P Notch Man Y/2(GenSpeedIN), Moving 3P Notch Man Y/2(GenSpeedIN), Moving 6P Notch Man Z/2(GenSpeedIN), Moving 3P Notch Man Z/2(GenSpeedIN)
  Mx/1 -> Mux/1, Moving 3P Notch Man Y/1(Input)
  My/1 -> Mux1/1, Moving 3P Notch Man Z/1(Input)
  Moving 6P Notch Man Z/1(Output) -> Discrete Filter3/1
  Moving 6P Notch Man Y/1(Output) -> Discrete Filter2/1
  Moving 3P Notch Man Y/1(Output) -> Moving 6P Notch Man Y/1(Input)
  Moving 3P Notch Man Z/1(Output) -> Moving 6P Notch Man Z/1(Input)
  Mux1/1 -> IPC NFs Man 2/2
  Mux/1 -> IPC NFs Man 2/1
  Discrete Filter3/1 -> Mux1/2, My_hat/1
  Discrete Filter2/1 -> Mux/2, Mx_hat/1

== system ROSCO/Monitor2/Cyclic Pitch controller/2P Cyclic Pitch Controller2/M0 Signal Proc.1 ==
  "My1,2, 3" : Inport
  GenSpeed : Inport  Port=2
  Add : Sum  Inputs=+++
  Demux1 : Demux  Outputs=3
  Discrete Filter : DiscreteFilter  Numerator=Parameter.Control.cIPC.PSM0_LPF.Numerator{1}  Denominator=Parameter.Control.cIPC.PSM0_LPF.Denominator{1}  a0EqualsOne=on
  Gain : Gain  Gain=1/3
  Moving 1P Notch Man : Subsystem
  Moving 3P Notch Man : Subsystem
  Mux : Mux  Inputs=2
  Scope : Scope  NumInputPorts=2
  M0 : Outport  VectorParamsAs1DForOutWhenUnconnected=off
  wires:
  Demux1/1 -> Add/1
  Demux1/2 -> Add/2
  Add/1 -> Gain/1
  "My1,2, 3"/1 -> Demux1/1
  GenSpeed/1 -> Moving 3P Notch Man/2(GenSpeedIN), Moving 1P Notch Man/2(GenSpeedIN)
  Demux1/3 -> Add/3
  Moving 1P Notch Man/1(Output) -> Moving 3P Notch Man/1(Input)
  Mux/1 -> Scope/2
  Gain/1 -> Scope/1, Moving 1P Notch Man/1(Input)
  Moving 3P Notch Man/1(Output) -> Discrete Filter/1
  Discrete Filter/1 -> Mux/1, M0/1

== system ROSCO/Monitor2/Cyclic Pitch controller/2P Cyclic Pitch Controller2/Norm ==
  In1 : Inport
  In2 : Inport  Port=2
  Add : Sum
  Discrete Filter1 : DiscreteFilter  Numerator=Parameter.Control.cIPC.IPCDQ_LPF.num{1}  Denominator=Parameter.Control.cIPC.IPCDQ_LPF.den{1}  SampleTime=Parameter.Control.DT
  Product : Product
  Product1 : Product
  Sqrt : Sqrt
  Out1 : Outport  VectorParamsAs1DForOutWhenUnconnected=off
  wires:
  Discrete Filter1/1 -> Out1/1
  In1/1 -> Product/2, Product/1
  In2/1 -> Product1/2, Product1/1
  Add/1 -> Sqrt/1
  Sqrt/1 -> Discrete Filter1/1
  Product1/1 -> Add/2
  Product/1 -> Add/1

== system ROSCO/Monitor2/Cyclic Pitch controller/2P Cyclic Pitch Controller2/Norm Pitch 2 ==
  b_dqsat : Inport
  Demux1 : Demux  Outputs=2
  Sqrt : Sqrt
  Square : Math  Operator=square  SignedPower=on
  Square1 : Math  Operator=square  SignedPower=on
  Sum : Sum
  Out1 : Outport  VectorParamsAs1DForOutWhenUnconnected=off
  wires:
  Sqrt/1 -> Out1/1
  Square/1 -> Sum/1
  Demux1/2 -> Square1/1
  Sum/1 -> Sqrt/1
  b_dqsat/1 -> Demux1/1
  Square1/1 -> Sum/2
  Demux1/1 -> Square/1

== system ROSCO/Monitor2/Cyclic Pitch controller/2P Cyclic Pitch Controller2/PI - D ==
  Md : Inport
  Anti-windup : Inport  Port=2
  Discrete Derivative : simulink/Discrete/Discrete Derivative  gainval=1.0  ICPrevScaledInput=0.0  OutMin=[]  OutMax=[]  OutDataType=fixdt(1, 16)  OutScaling=2^-10  DoSatur=off
  Discrete Filter1 : DiscreteFilter  Commented=through  Numerator=Parameter.Control.cIPC.IPCDQ_LPF.num{1}  Denominator=Parameter.Control.cIPC.IPCDQ_LPF.den{1}  SampleTime=Parameter.Control.DT
  Integrator : DiscreteIntegrator  IntegratorMethod=Integration: Backward Euler  gainval=1  SampleTime=simu.dt  UpperSaturationLimit=1.570796/(.008068634/9.5492966)/(1./(1.+pi/2/.109997))  LowerSaturationLimit=0  ICPrevOutput=DiscIntNeverNeededParam  ICPrevScaledInput=DiscIntNeverNeededParam
  Kd : Gain  Gain=0
  Ki : Gain  Gain=R.IPC_KI_2P
  Kp : Gain  Gain=R.IPC_KP_2P
  Sum3 : Sum  Inputs=+++
  Sum8 : Sum  Inputs=|++
  Theta_tilt : Outport  VectorParamsAs1DForOutWhenUnconnected=off
  wires:
  Discrete Filter1/1 -> Kd/1
  Integrator/1 -> Sum3/3
  Discrete Derivative/1 -> Sum3/1
  Kp/1 -> Sum3/2
  Kd/1 -> Discrete Derivative/1
  Sum8/1 -> Integrator/1
  Anti-windup/1 -> Sum8/2
  Md/1 -> Discrete Filter1/1, Kp/1, Ki/1
  Sum3/1 -> Theta_tilt/1
  Ki/1 -> Sum8/1

== system ROSCO/Monitor2/Cyclic Pitch controller/2P Cyclic Pitch Controller2/PI - Q ==
  Mq : Inport
  Anti-windup : Inport  Port=2
  Discrete Derivative : simulink/Discrete/Discrete Derivative  gainval=1.0  ICPrevScaledInput=0.0  OutMin=[]  OutMax=[]  OutDataType=fixdt(1, 16)  OutScaling=2^-10  DoSatur=off
  Discrete Filter1 : DiscreteFilter  Commented=through  Numerator=Parameter.Control.cIPC.IPCDQ_LPF.num{1}  Denominator=Parameter.Control.cIPC.IPCDQ_LPF.den{1}  SampleTime=Parameter.Control.DT
  Integrator1 : DiscreteIntegrator  IntegratorMethod=Integration: Backward Euler  gainval=1  SampleTime=simu.dt  UpperSaturationLimit=1.570796/(.008068634/9.5492966)/(1./(1.+pi/2/.109997))  LowerSaturationLimit=0  ICPrevOutput=DiscIntNeverNeededParam  ICPrevScaledInput=DiscIntNeverNeededParam
  Kd : Gain  Gain=0
  Ki : Gain  Gain=R.IPC_KI_2P
  Kp : Gain  Gain=R.IPC_KP_2P
  Sum10 : Sum  Inputs=|++
  Sum3 : Sum  Inputs=+++
  Theta_yaw : Outport  VectorParamsAs1DForOutWhenUnconnected=off
  wires:
  Discrete Filter1/1 -> Kd/1
  Discrete Derivative/1 -> Sum3/1
  Kd/1 -> Discrete Derivative/1
  Mq/1 -> Ki/1, Kp/1, Discrete Filter1/1
  Kp/1 -> Sum3/2
  Ki/1 -> Sum10/1
  Integrator1/1 -> Sum3/3
  Anti-windup/1 -> Sum10/2
  Sum10/1 -> Integrator1/1
  Sum3/1 -> Theta_yaw/1

== system ROSCO/Monitor2/Cyclic Pitch controller/2P Cyclic Pitch Controller2/Subsystem ==
  Constant3 : Constant
  Constant4 : Constant  Value=0
  Constant5 : Constant  Value=0
  Mux : Mux  Inputs=3
  IPC Sat Params : Outport  VectorParamsAs1DForOutWhenUnconnected=off
  wires:
  Constant3/1 -> Mux/1
  Constant4/1 -> Mux/2
  Constant5/1 -> Mux/3
  Mux/1 -> IPC Sat Params/1

== system ROSCO/Monitor2/Cyclic Pitch controller/1P Cyclic Pitch Controller1/1P IPCDQ Filtering1/Moving 3P Notch Man Y ==
  Input : Inport
  GenSpeedIN : Inport  Port=2
  Gain : Gain  Gain=1/Parameter.Turbine.G * rpm2radps(1) * 3
  Moving 3P Filt Manual : Subsystem
  Slow Low Pass for Param : DiscreteStateSpace  A=Parameter.Control.cIPC.dLPF_slow.a  B=Parameter.Control.cIPC.dLPF_slow.b  C=Parameter.Control.cIPC.dLPF_slow.c  D=Parameter.Control.cIPC.dLPF_slow.d  SampleTime=Parameter.Control.DT
  Output : Outport  VectorParamsAs1DForOutWhenUnconnected=off
  wires:
  Slow Low Pass for Param/1 -> Gain/1
  Gain/1 -> Moving 3P Filt Manual/2(rot speed (rad/s))
  Input/1 -> Moving 3P Filt Manual/1(u)
  GenSpeedIN/1 -> Slow Low Pass for Param/1
  Moving 3P Filt Manual/1(Out1) -> Output/1

== system ROSCO/Monitor2/Cyclic Pitch controller/1P Cyclic Pitch Controller1/1P IPCDQ Filtering1/Moving 3P Notch Man Z ==
  Input : Inport
  GenSpeedIN : Inport  Port=2
  Gain : Gain  Gain=1/Parameter.Turbine.G * rpm2radps(1) * 3
  Moving 3P Filt Manual : Subsystem
  Slow Low Pass for Param : DiscreteStateSpace  A=Parameter.Control.cIPC.dLPF_slow.a  B=Parameter.Control.cIPC.dLPF_slow.b  C=Parameter.Control.cIPC.dLPF_slow.c  D=Parameter.Control.cIPC.dLPF_slow.d  SampleTime=Parameter.Control.DT
  Output : Outport  VectorParamsAs1DForOutWhenUnconnected=off
  wires:
  Moving 3P Filt Manual/1(Out1) -> Output/1
  GenSpeedIN/1 -> Slow Low Pass for Param/1
  Input/1 -> Moving 3P Filt Manual/1(u)
  Gain/1 -> Moving 3P Filt Manual/2(rot speed (rad/s))
  Slow Low Pass for Param/1 -> Gain/1

== system ROSCO/Monitor2/Cyclic Pitch controller/1P Cyclic Pitch Controller1/1P IPCDQ Filtering1/Moving 6P Notch Man Y ==
  Input : Inport
  GenSpeedIN : Inport  Port=2
  Gain : Gain  Gain=1/Parameter.Turbine.G * rpm2radps(1) * 3
  Moving 6P Filt Manual : Subsystem
  Slow Low Pass for Param : DiscreteStateSpace  A=Parameter.Control.cIPC.dLPF_slow.a  B=Parameter.Control.cIPC.dLPF_slow.b  C=Parameter.Control.cIPC.dLPF_slow.c  D=Parameter.Control.cIPC.dLPF_slow.d  SampleTime=Parameter.Control.DT
  Output : Outport  VectorParamsAs1DForOutWhenUnconnected=off
  wires:
  Moving 6P Filt Manual/1(Out1) -> Output/1
  GenSpeedIN/1 -> Slow Low Pass for Param/1
  Input/1 -> Moving 6P Filt Manual/1(u)
  Gain/1 -> Moving 6P Filt Manual/2(rot speed (rad/s))
  Slow Low Pass for Param/1 -> Gain/1

== system ROSCO/Monitor2/Cyclic Pitch controller/1P Cyclic Pitch Controller1/1P IPCDQ Filtering1/Moving 6P Notch Man Z ==
  Input : Inport
  GenSpeedIN : Inport  Port=2
  Gain : Gain  Gain=1/Parameter.Turbine.G * rpm2radps(1) * 3
  Moving 6P Filt Manual : Subsystem
  Slow Low Pass for Param : DiscreteStateSpace  A=Parameter.Control.cIPC.dLPF_slow.a  B=Parameter.Control.cIPC.dLPF_slow.b  C=Parameter.Control.cIPC.dLPF_slow.c  D=Parameter.Control.cIPC.dLPF_slow.d  SampleTime=Parameter.Control.DT
  Output : Outport  VectorParamsAs1DForOutWhenUnconnected=off
  wires:
  Slow Low Pass for Param/1 -> Gain/1
  Gain/1 -> Moving 6P Filt Manual/2(rot speed (rad/s))
  Input/1 -> Moving 6P Filt Manual/1(u)
  GenSpeedIN/1 -> Slow Low Pass for Param/1
  Moving 6P Filt Manual/1(Out1) -> Output/1

== system ROSCO/Monitor2/Cyclic Pitch controller/1P Cyclic Pitch Controller1/M0 Signal Proc.1/Moving 1P Notch Man ==
  Input : Inport
  GenSpeedIN : Inport  Port=2
  Gain : Gain  Gain=1/Parameter.Turbine.G * rpm2radps(1)
  Moving 1P Filt Manual : Subsystem
  Slow Low Pass for Param : DiscreteStateSpace  A=Parameter.Control.cIPC.dLPF_slow.a  B=Parameter.Control.cIPC.dLPF_slow.b  C=Parameter.Control.cIPC.dLPF_slow.c  D=Parameter.Control.cIPC.dLPF_slow.d  SampleTime=Parameter.Control.DT
  Output : Outport  VectorParamsAs1DForOutWhenUnconnected=off
  wires:
  GenSpeedIN/1 -> Slow Low Pass for Param/1
  Input/1 -> Moving 1P Filt Manual/1(u)
  Gain/1 -> Moving 1P Filt Manual/2(rot speed (rad/s))
  Slow Low Pass for Param/1 -> Gain/1
  Moving 1P Filt Manual/1(Out1) -> Output/1

== system ROSCO/Monitor2/Cyclic Pitch controller/1P Cyclic Pitch Controller1/M0 Signal Proc.1/Moving 3P Notch Man ==
  Input : Inport
  GenSpeedIN : Inport  Port=2
  Gain : Gain  Gain=1/Parameter.Turbine.G * rpm2radps(1) * 3
  Moving 3P Filt Manual : Subsystem
  Slow Low Pass for Param : DiscreteStateSpace  A=Parameter.Control.cIPC.dLPF_slow.a  B=Parameter.Control.cIPC.dLPF_slow.b  C=Parameter.Control.cIPC.dLPF_slow.c  D=Parameter.Control.cIPC.dLPF_slow.d  SampleTime=Parameter.Control.DT
  Output : Outport  VectorParamsAs1DForOutWhenUnconnected=off
  wires:
  Slow Low Pass for Param/1 -> Gain/1
  Gain/1 -> Moving 3P Filt Manual/2(rot speed (rad/s))
  Input/1 -> Moving 3P Filt Manual/1(u)
  GenSpeedIN/1 -> Slow Low Pass for Param/1
  Moving 3P Filt Manual/1(Out1) -> Output/1

== system ROSCO/Monitor2/Cyclic Pitch controller/2P Cyclic Pitch Controller2/1P IPCDQ Filtering1/Moving 3P Notch Man Y ==
  Input : Inport
  GenSpeedIN : Inport  Port=2
  Gain : Gain  Gain=1/Parameter.Turbine.G * rpm2radps(1) * 3
  Moving 3P Filt Manual : Subsystem
  Slow Low Pass for Param : DiscreteStateSpace  A=Parameter.Control.cIPC.dLPF_slow.a  B=Parameter.Control.cIPC.dLPF_slow.b  C=Parameter.Control.cIPC.dLPF_slow.c  D=Parameter.Control.cIPC.dLPF_slow.d  SampleTime=Parameter.Control.DT
  Output : Outport  VectorParamsAs1DForOutWhenUnconnected=off
  wires:
  Slow Low Pass for Param/1 -> Gain/1
  Gain/1 -> Moving 3P Filt Manual/2(rot speed (rad/s))
  Input/1 -> Moving 3P Filt Manual/1(u)
  GenSpeedIN/1 -> Slow Low Pass for Param/1
  Moving 3P Filt Manual/1(Out1) -> Output/1

== system ROSCO/Monitor2/Cyclic Pitch controller/2P Cyclic Pitch Controller2/1P IPCDQ Filtering1/Moving 3P Notch Man Z ==
  Input : Inport
  GenSpeedIN : Inport  Port=2
  Gain : Gain  Gain=1/Parameter.Turbine.G * rpm2radps(1) * 3
  Moving 3P Filt Manual : Subsystem
  Slow Low Pass for Param : DiscreteStateSpace  A=Parameter.Control.cIPC.dLPF_slow.a  B=Parameter.Control.cIPC.dLPF_slow.b  C=Parameter.Control.cIPC.dLPF_slow.c  D=Parameter.Control.cIPC.dLPF_slow.d  SampleTime=Parameter.Control.DT
  Output : Outport  VectorParamsAs1DForOutWhenUnconnected=off
  wires:
  Moving 3P Filt Manual/1(Out1) -> Output/1
  GenSpeedIN/1 -> Slow Low Pass for Param/1
  Input/1 -> Moving 3P Filt Manual/1(u)
  Gain/1 -> Moving 3P Filt Manual/2(rot speed (rad/s))
  Slow Low Pass for Param/1 -> Gain/1

== system ROSCO/Monitor2/Cyclic Pitch controller/2P Cyclic Pitch Controller2/1P IPCDQ Filtering1/Moving 6P Notch Man Y ==
  Input : Inport
  GenSpeedIN : Inport  Port=2
  Gain : Gain  Gain=1/Parameter.Turbine.G * rpm2radps(1) * 3
  Moving 6P Filt Manual : Subsystem
  Slow Low Pass for Param : DiscreteStateSpace  A=Parameter.Control.cIPC.dLPF_slow.a  B=Parameter.Control.cIPC.dLPF_slow.b  C=Parameter.Control.cIPC.dLPF_slow.c  D=Parameter.Control.cIPC.dLPF_slow.d  SampleTime=Parameter.Control.DT
  Output : Outport  VectorParamsAs1DForOutWhenUnconnected=off
  wires:
  Moving 6P Filt Manual/1(Out1) -> Output/1
  GenSpeedIN/1 -> Slow Low Pass for Param/1
  Input/1 -> Moving 6P Filt Manual/1(u)
  Gain/1 -> Moving 6P Filt Manual/2(rot speed (rad/s))
  Slow Low Pass for Param/1 -> Gain/1

== system ROSCO/Monitor2/Cyclic Pitch controller/2P Cyclic Pitch Controller2/1P IPCDQ Filtering1/Moving 6P Notch Man Z ==
  Input : Inport
  GenSpeedIN : Inport  Port=2
  Gain : Gain  Gain=1/Parameter.Turbine.G * rpm2radps(1) * 3
  Moving 6P Filt Manual : Subsystem
  Slow Low Pass for Param : DiscreteStateSpace  A=Parameter.Control.cIPC.dLPF_slow.a  B=Parameter.Control.cIPC.dLPF_slow.b  C=Parameter.Control.cIPC.dLPF_slow.c  D=Parameter.Control.cIPC.dLPF_slow.d  SampleTime=Parameter.Control.DT
  Output : Outport  VectorParamsAs1DForOutWhenUnconnected=off
  wires:
  Slow Low Pass for Param/1 -> Gain/1
  Gain/1 -> Moving 6P Filt Manual/2(rot speed (rad/s))
  Input/1 -> Moving 6P Filt Manual/1(u)
  GenSpeedIN/1 -> Slow Low Pass for Param/1
  Moving 6P Filt Manual/1(Out1) -> Output/1

== system ROSCO/Monitor2/Cyclic Pitch controller/2P Cyclic Pitch Controller2/M0 Signal Proc.1/Moving 1P Notch Man ==
  Input : Inport
  GenSpeedIN : Inport  Port=2
  Gain : Gain  Gain=1/Parameter.Turbine.G * rpm2radps(1)
  Moving 1P Filt Manual : Subsystem
  Slow Low Pass for Param : DiscreteStateSpace  A=Parameter.Control.cIPC.dLPF_slow.a  B=Parameter.Control.cIPC.dLPF_slow.b  C=Parameter.Control.cIPC.dLPF_slow.c  D=Parameter.Control.cIPC.dLPF_slow.d  SampleTime=Parameter.Control.DT
  Output : Outport  VectorParamsAs1DForOutWhenUnconnected=off
  wires:
  GenSpeedIN/1 -> Slow Low Pass for Param/1
  Input/1 -> Moving 1P Filt Manual/1(u)
  Gain/1 -> Moving 1P Filt Manual/2(rot speed (rad/s))
  Slow Low Pass for Param/1 -> Gain/1
  Moving 1P Filt Manual/1(Out1) -> Output/1

== system ROSCO/Monitor2/Cyclic Pitch controller/2P Cyclic Pitch Controller2/M0 Signal Proc.1/Moving 3P Notch Man ==
  Input : Inport
  GenSpeedIN : Inport  Port=2
  Gain : Gain  Gain=1/Parameter.Turbine.G * rpm2radps(1) * 3
  Moving 3P Filt Manual : Subsystem
  Slow Low Pass for Param : DiscreteStateSpace  A=Parameter.Control.cIPC.dLPF_slow.a  B=Parameter.Control.cIPC.dLPF_slow.b  C=Parameter.Control.cIPC.dLPF_slow.c  D=Parameter.Control.cIPC.dLPF_slow.d  SampleTime=Parameter.Control.DT
  Output : Outport  VectorParamsAs1DForOutWhenUnconnected=off
  wires:
  Slow Low Pass for Param/1 -> Gain/1
  Gain/1 -> Moving 3P Filt Manual/2(rot speed (rad/s))
  Input/1 -> Moving 3P Filt Manual/1(u)
  GenSpeedIN/1 -> Slow Low Pass for Param/1
  Moving 3P Filt Manual/1(Out1) -> Output/1

== system ROSCO/Monitor2/Cyclic Pitch controller/1P Cyclic Pitch Controller1/1P IPCDQ Filtering1/Moving 3P Notch Man Y/Moving 3P Filt Manual ==
  u : Inport
  rot speed (rad/s) : Inport  Port=2
  Den LPV : Subsystem
  Discrete Filter : DiscreteFilter  NumeratorSource=Input port  DenominatorSource=Input port  a0EqualsOne=on
      settings: InputPortMap=u0,p1,p3
  Num LPV : Subsystem
  Out1 : Outport  VectorParamsAs1DForOutWhenUnconnected=off
  wires:
  u/1 -> Discrete Filter/1
  Num LPV/1(b) -> Discrete Filter/2
  Discrete Filter/1 -> Out1/1
  rot speed (rad/s)/1 -> Den LPV/1(rot speed (rad/s)), Num LPV/1(rot speed (rad/s))
  Den LPV/1(a) -> Discrete Filter/3
